simulink library "mylib"  (R2019b)
settings: Solver=VariableStepAuto  StartTime=0.0  StopTime=10.0  RelTol=1e-3
undefined symbols (not defined in the file or in its folder): AG, AH, AV, BCHL, BCHV, BG, BH, CG, CH, magnitude, Ts, XMW
libraries: $bdroot x28, TElib x2
(part 2 of 3)

== system mylib/Process Noise I=1-12 G New/TESUB6 ==
  STD : Inport
  G : Inport  Port=2
  Constant : Constant  Value=6
  Product : Product
  Subsystem : Subsystem
  Subtract : Sum  Inputs=+-
  X : Outport  VectorParamsAs1DForOutWhenUnconnected=off
  G_NEW : Outport  Port=2  VectorParamsAs1DForOutWhenUnconnected=off
  wires:
  STD/1 -> Product/2
  Product/1 -> X/1
  Subtract/1 -> Product/1
  Constant/1 -> Subtract/2
  G/1 -> Subsystem/1(G)
  Subsystem/1(TESUB7) -> Subtract/1
  Subsystem/2(G_NEW) -> G_NEW/1

== system mylib/Process Noise I=1-22/If Action Subsystem ==
  In1 : Inport
  Action Port : ActionPort
  Out1 : Outport  VectorParamsAs1DForOutWhenUnconnected=off
  wires:
  In1/1 -> Out1/1

== system mylib/Process Noise I=23-36/Gas Analysis Delay ==
  Clock : Clock
  Constant : Constant  Value=3600
  If : If  IfExpression=u1 == 0  ShowElse=off
  Math Function : Math  Operator=mod  SaturateOnIntegerOverflow=on
  Merge : Merge
  Product : Product
  Subsystem : Subsystem
      mask Display: color('Blue'), disp('MOD\nFix');
  TGAS Delay 0.1h : Constant  Value=360
  IF(TGAS) : Outport  VectorParamsAs1DForOutWhenUnconnected=off
  wires:
  Math Function/1 -> Subsystem/1(In1)
  Subsystem/2(Out2) -> Merge/2
  Subsystem/1(Out1) -> Merge/1
  Merge/1 -> If/1
  Constant/1 -> Product/2
  If/1 -> IF(TGAS)/1
  Clock/1 -> Product/1
  TGAS Delay 0.1h/1 -> Math Function/2, Subsystem/2(In2)
  Product/1 -> Math Function/1

== system mylib/Process Noise I=23-36/If Action Subsystem ==
  XCMP : Inport
  XDEL_OLD : Inport  Port=2
  XMNS : Inport  Port=3
  Action Port : ActionPort
  Add : Sum
  XDEL_NEW : Outport  VectorParamsAs1DForOutWhenUnconnected=off
  XMEAS : Outport  Port=2  VectorParamsAs1DForOutWhenUnconnected=off
  wires:
  XCMP/1 -> XDEL_NEW/1
  Add/1 -> XMEAS/1
  XDEL_OLD/1 -> Add/1
  XMNS/1 -> Add/2

== system mylib/Process Noise I=23-36/If Action Subsystem1 ==
  In1 : Inport
  Action Port : ActionPort
  Out1 : Outport  VectorParamsAs1DForOutWhenUnconnected=off
  wires:
  In1/1 -> Out1/1

== system mylib/Process Noise I=37-41/Gas Analysis Delay ==
  Clock : Clock
  Constant : Constant  Value=3600
  If : If  IfExpression=u1 == 0  ShowElse=off
  Math Function : Math  Operator=mod  SaturateOnIntegerOverflow=on
  Merge : Merge
  Product : Product
  Subsystem : Subsystem
      mask Display: color('Blue'), disp('MOD\nFix');
  TPROD Delay 0.25h : Constant  Value=900
  IF(TPROD) : Outport  VectorParamsAs1DForOutWhenUnconnected=off
  wires:
  Merge/1 -> If/1
  Subsystem/2(Out2) -> Merge/2
  Subsystem/1(Out1) -> Merge/1
  Math Function/1 -> Subsystem/1(In1)
  Constant/1 -> Product/2
  If/1 -> IF(TPROD)/1
  Clock/1 -> Product/1
  TPROD Delay 0.25h/1 -> Math Function/2, Subsystem/2(In2)
  Product/1 -> Math Function/1

== system mylib/Process Noise I=37-41/If Action Subsystem ==
  XCMP : Inport
  XDEL_OLD : Inport  Port=2
  XMNS : Inport  Port=3
  Action Port : ActionPort
  Add : Sum
  XDEL_NEW : Outport  VectorParamsAs1DForOutWhenUnconnected=off
  XMEAS : Outport  Port=2  VectorParamsAs1DForOutWhenUnconnected=off
  wires:
  XCMP/1 -> XDEL_NEW/1
  Add/1 -> XMEAS/1
  XDEL_OLD/1 -> Add/1
  XMNS/1 -> Add/2

== system mylib/Subsystem3/If Action Subsystem ==
  IDWLK : Inport
  "DIST " : Inport  Port=2
  G : Inport  Port=3
  Distrubance constants : Inport  Port=4
  Action Port : ActionPort
  Bus Creator : BusCreator  Inputs=6
  Bus Selector : BusSelector  OutputSignals=ADIST,BDIST,CDIST,DDIST,TNEXT,TLAST
  Disturbance parameters I=10-12 : Subsystem
      mask Display:
      | color('Green'), disp('Disturbance parameters\n I=10-12');
      | color('Blue');
      | port_label('input',1,'ADIST');
      | port_label('input',2,'BDIST');
      | port_label('input',3,'CDIST');
      | port_label('input',4,'DDIST');
      | port_label('input',5,'TNEXT');
      | port_label('input',6,'TLAST');
      | port_label('input',7,'IDVWLK');
      | port_label('input',8,'Distrubance constants');
      | port_label('input',9,'G');
      | port_label('output',1,'ADIST');
      | port_label('output',2,'BDIST');
      | port_label('output',3,'CDIST');
      | port_label('output',4,'DDIST');
      | port_label('output',5,'TNEXT');
      | port_label('output',6,'TLAST');
      | port_label('output',7,'G_NEW');
  DIST_NEW : Outport  PortDimensions=6  VectorParamsAs1DForOutWhenUnconnected=off
  "G_NEW " : Outport  Port=2  VectorParamsAs1DForOutWhenUnconnected=off
  wires:
  Disturbance parameters I=10-12/5("TNEXT ") -> Bus Creator/5  "TNEXT"
  Bus Creator/1 -> DIST_NEW/1
  IDWLK/1 -> Disturbance parameters I=10-12/7(IDVWLK)
  Bus Selector/1 -> Disturbance parameters I=10-12/1(ADIST)  "<ADIST>"
  Distrubance constants/1 -> Disturbance parameters I=10-12/8(Distrubance constants)
  Bus Selector/2 -> Disturbance parameters I=10-12/2(BDIST)  "<BDIST>"
  Disturbance parameters I=10-12/1("ADIST ") -> Bus Creator/1  "ADIST"
  Bus Selector/6 -> Disturbance parameters I=10-12/6(TLAST)  "<TLAST>"
  Bus Selector/5 -> Disturbance parameters I=10-12/5(TNEXT)  "<TNEXT>"
  Disturbance parameters I=10-12/4("DDIST ") -> Bus Creator/4  "DDIST"
  Disturbance parameters I=10-12/3("CDIST ") -> Bus Creator/3  "CDIST"
  Bus Selector/4 -> Disturbance parameters I=10-12/4(DDIST)  "<DDIST>"
  Disturbance parameters I=10-12/6("TLAST  ") -> Bus Creator/6  "TLAST"
  Bus Selector/3 -> Disturbance parameters I=10-12/3(CDIST)  "<CDIST>"
  "DIST "/1 -> Bus Selector/1
  Disturbance parameters I=10-12/2("BDIST ") -> Bus Creator/2  "BDIST"
  G/1 -> Disturbance parameters I=10-12/9(G)
  Disturbance parameters I=10-12/7("G_NEW ") -> "G_NEW "/1  "G_NEW"

== system mylib/Subsystem3/If Action Subsystem1 ==
  DIST_0 : Inport
  Action Port : ActionPort
  DIST : Outport  VectorParamsAs1DForOutWhenUnconnected=off
  wires:
  DIST_0/1 -> DIST/1

== system mylib/Subsystem3/Subsystem ==
  TNEXT : Inport
  Clock : Clock
  Constant : Constant  Value=3600
  Data Type Conversion : DataTypeConversion  OutDataTypeStr=double
  If : If  NumInputs=2  IfExpression=u1 == 0  ElseIfExpressions=u1 >= u2  ShowElse=off
  Product : Product
  Product1 : Product  OutDataTypeStr=fixdt(1,32,10)
  if : Outport
  elseif : Outport  Port=2
  wires:
  Data Type Conversion/1 -> If/2
  Product1/1 -> Data Type Conversion/1
  TNEXT/1 -> Product1/2
  Product/1 -> If/1
  Clock/1 -> Product/1
  Constant/1 -> Product/2, Product1/1
  If/1 -> if/1
  If/2 -> elseif/1

== system mylib/Subsystem3/Subsystem1 ==
  DIST_NEW : Inport
  Bus Creator : BusCreator  Inputs=6
  Bus Selector : BusSelector  OutputSignals=ADIST,BDIST,CDIST,DDIST,TNEXT,TLAST
  Delay{,1..5} (6 alike) : Delay  DelayLength=1  InitialCondition=0
  DIST : Outport
  wires:
  DIST_NEW/1 -> Bus Selector/1
  Bus Creator/1 -> DIST/1
  Delay/1 -> Bus Creator/1  "ADIST"
  Delay3/1 -> Bus Creator/4  "DDIST"
  Bus Selector/5 -> Delay4/1  "<TNEXT>"
  Delay4/1 -> Bus Creator/5  "TNEXT"
  Bus Selector/4 -> Delay3/1  "<DDIST>"
  Bus Selector/2 -> Delay1/1  "<BDIST>"
  Delay2/1 -> Bus Creator/3  "CDIST"
  Bus Selector/3 -> Delay2/1  "<CDIST>"
  Delay5/1 -> Bus Creator/6  "TLAST"
  Delay1/1 -> Bus Creator/2  "BDIST"
  Bus Selector/6 -> Delay5/1  "<TLAST>"
  Bus Selector/1 -> Delay/1  "<ADIST>"

== system mylib/Subsystem3/Subsystem2 ==
  In2 : Inport
  G : Inport  Port=2
  If Action Subsystem : Subsystem  TreatAsAtomicUnit=on
  If Action Subsystem1 : Subsystem  TreatAsAtomicUnit=on
  If5 : If  IfExpression=u1 == 0
  Merge : Merge
  G1 : Outport  VectorParamsAs1DForOutWhenUnconnected=off
  wires:
  In2/1 -> If Action Subsystem1/1(In1), If5/1
  If5/2 -> If Action Subsystem1/Action
  If Action Subsystem1/1(Out1) -> Merge/1
  If5/1 -> If Action Subsystem/Action
  If Action Subsystem/1(Out1) -> Merge/2
  G/1 -> If Action Subsystem/1(In1)
  Merge/1 -> G1/1

== system mylib/TESUB5/Subsystem ==
  TESUB7 : Inport
  HSPAN : Inport  Port=2
  HZERO : Inport  Port=3
  H : Sum
  Product : Product
  "H " : Outport  VectorParamsAs1DForOutWhenUnconnected=off
  wires:
  H/1 -> "H "/1
  Product/1 -> H/1
  HSPAN/1 -> Product/1
  HZERO/1 -> H/2
  TESUB7/1 -> Product/2

== system mylib/TESUB5/Subsystem1 ==
  SSPAN : Inport
  TESUB7 : Inport  Port=2
  SZERO : Inport  Port=3
  IDVFLAG : Inport  Port=4
  Product1 : Product  Inputs=3
  S1 : Sum
  "S1 " : Outport  VectorParamsAs1DForOutWhenUnconnected=off
  wires:
  SZERO/1 -> S1/2
  Product1/1 -> S1/1
  S1/1 -> "S1 "/1
  IDVFLAG/1 -> Product1/3
  TESUB7/1 -> Product1/2
  SSPAN/1 -> Product1/1

== system mylib/TESUB5/Subsystem2 ==
  TESUB7 : Inport
  SPSPAN : Inport  Port=2
  IDVFLAG : Inport  Port=3
  S1P : Product  Inputs=3
  "S1P " : Outport  VectorParamsAs1DForOutWhenUnconnected=off
  wires:
  IDVFLAG/1 -> S1P/3
  S1P/1 -> "S1P "/1
  TESUB7/1 -> S1P/2
  SPSPAN/1 -> S1P/1

== system mylib/TESUB5/Subsystem3 ==
  SP : Inport
  S1 : Inport  Port=2
  S : Inport  Port=3
  S1P : Inport  Port=4
  H : Inport  Port=5
  Add1 : Sum
  Constant : Constant  Value=3
  Constant1 : Constant  Value=2
  Divide : Product  Inputs=*/
  Math Function : Math  Operator=magnitude^2  SaturateOnIntegerOverflow=on
  Product2 : Product
  Product3 : Product
  Product4 : Product
  Subtract : Sum  Inputs=+-
  Subtract1 : Sum  Inputs=+-
  CDIST : Outport  VectorParamsAs1DForOutWhenUnconnected=off
  wires:
  Product3/1 -> Add1/2
  Subtract1/1 -> Divide/1
  Product4/1 -> Subtract1/2
  Math Function/1 -> Divide/2
  Product2/1 -> Subtract1/1
  S1/1 -> Subtract/1
  Constant/1 -> Product2/2
  SP/1 -> Product3/1
  Constant1/1 -> Product3/2
  Add1/1 -> Product4/2
  Subtract/1 -> Product2/1
  Divide/1 -> CDIST/1
  S/1 -> Subtract/2
  H/1 -> Product4/1, Math Function/1
  S1P/1 -> Add1/1

== system mylib/TESUB5/Subsystem4 ==
  SP : Inport
  S1 : Inport  Port=2
  S : Inport  Port=3
  S1P : Inport  Port=4
  H : Inport  Port=5
  Add2 : Sum
  Add3 : Sum
  Constant : Constant  Value=3
  Constant1 : Constant  Value=2
  Divide1 : Product  Inputs=*/
  Math Function1 : Math  Operator=pow  SaturateOnIntegerOverflow=on
  Product5 : Product
  Product6 : Product
  Subtract2 : Sum  Inputs=+-
  DDIST : Outport  VectorParamsAs1DForOutWhenUnconnected=off
  wires:
  Product5/1 -> Add3/1
  Divide1/1 -> DDIST/1
  SP/1 -> Add2/2
  Product6/1 -> Add3/2
  S/1 -> Subtract2/1
  Add2/1 -> Product6/2
  Math Function1/1 -> Divide1/2
  Subtract2/1 -> Product5/1
  Constant/1 -> Math Function1/2
  Add3/1 -> Divide1/1
  H/1 -> Product6/1, Math Function1/1
  S1/1 -> Subtract2/2
  S1P/1 -> Add2/1
  Constant1/1 -> Product5/2

== system mylib/TESUB5/Subsystem5 ==
  TLAST : Inport
  H : Inport  Port=2
  Add : Sum
  TNEXT : Outport  VectorParamsAs1DForOutWhenUnconnected=off
  wires:
  Add/1 -> TNEXT/1
  TLAST/1 -> Add/1
  H/1 -> Add/2

== system mylib/TESUB6/TESUB7 ==
  G : Inport
  I : Inport  Port=2
  Constant1 : Constant  Value=4294967296
  Divide : Product  Inputs=*/
  Divide1 : Product  Inputs=*/
  Gain : Gain  Gain=9228907
  New G : Math  Operator=rem  SaturateOnIntegerOverflow=on
  Product : Product
  Sum of Elements : Sum  Inputs=+
  TESUB7 : Outport  VectorParamsAs1DForOutWhenUnconnected=off
  wires:
  G/1 -> Gain/1
  Gain/1 -> New G/1
  Constant1/1 -> Divide/2, New G/2
  New G/1 -> Divide/1
  I/1 -> Divide1/2, Divide1/1
  Divide/1 -> Product/2
  Divide1/1 -> Product/1
  Product/1 -> Sum of Elements/1
  Sum of Elements/1 -> TESUB7/1

== system mylib/TESUB7/If Action Subsystem ==
  In1 : Inport
  Action Port : ActionPort
  Out1 : Outport  VectorParamsAs1DForOutWhenUnconnected=off
  wires:
  In1/1 -> Out1/1

== system mylib/TESUB7/If Action Subsystem1 ==
  In1 : Inport
  Action Port : ActionPort
  Out1 : Outport  VectorParamsAs1DForOutWhenUnconnected=off
  wires:
  In1/1 -> Out1/1

== system mylib/TESUB7 G-New/If Action Subsystem ==
  In1 : Inport
  Action Port : ActionPort
  Out1 : Outport  VectorParamsAs1DForOutWhenUnconnected=off
  wires:
  In1/1 -> Out1/1

== system mylib/TESUB7 G-New/If Action Subsystem1 ==
  In1 : Inport
  Action Port : ActionPort
  Out1 : Outport  VectorParamsAs1DForOutWhenUnconnected=off
  wires:
  In1/1 -> Out1/1

== system mylib/Valve opening limits/If Action Subsystem ==
  In1 : Inport
  Action Port : ActionPort
  Out1 : Outport  VectorParamsAs1DForOutWhenUnconnected=off
  wires:
  In1/1 -> Out1/1

== system mylib/Valve opening limits/If Action Subsystem1 ==
  In1 : Inport
  Action Port : ActionPort
  Out1 : Outport  VectorParamsAs1DForOutWhenUnconnected=off
  wires:
  In1/1 -> Out1/1

== system mylib/Valve opening limits/If Action Subsystem2 ==
  In1 : Inport
  Action Port : ActionPort
  Out1 : Outport  VectorParamsAs1DForOutWhenUnconnected=off
  wires:
  In1/1 -> Out1/1

== system mylib/Braatz Control/P Control/  ==
  DXMV : Inport
  XMV_0 : Inport  Port=2
  Add : Sum
  Delay : Delay  DelayLength=1  InitialConditionSource=Input port  InitialCondition=0
      settings: InputPortMap=u0,p4
  Subsystem1 : $bdroot/Braatz Control/Subsystem1  SystemSampleTime=-1  Latency=0  AutoFrameSizeCalculation=off
  XMV : Outport
  wires:
  XMV_0/1 -> Delay/2
  Delay/1 -> Add/1
  Add/1 -> Subsystem1/1
  Subsystem1/1 -> XMV/1, Delay/1
  DXMV/1 -> Add/2

== system mylib/Braatz Control/P Control/ERR ==
  SETPT : Inport
  XMEAS : Inport  Port=2
  High Limit : Inport  Port=3
  " " : Product  Inputs=**/
  Constant : Constant  Value=100
  Subtract : Sum  Inputs=+-
  ERR : Outport  VectorParamsAs1DForOutWhenUnconnected=off
  wires:
  Constant/1 -> " "/2
  High Limit/1 -> " "/3
  Subtract/1 -> " "/1
  SETPT/1 -> Subtract/1
  " "/1 -> ERR/1
  XMEAS/1 -> Subtract/2

== system mylib/Braatz Control/P Control/Subsystem ==
  ERR : Inport
  GAIN : Inport  Port=2
  ERROLD : Inport  Port=3
  Product : Product
  Subtract1 : Sum  Inputs=+-
  DXMV : Outport  VectorParamsAs1DForOutWhenUnconnected=off
  wires:
  GAIN/1 -> Product/1
  Product/1 -> DXMV/1
  Subtract1/1 -> Product/2
  ERROLD/1 -> Subtract1/2
  ERR/1 -> Subtract1/1

== system mylib/Braatz Control/PI Control/ERR ==
  SETPT : Inport
  XMEAS : Inport  Port=2
  High Limit : Inport  Port=3
  " " : Product  Inputs=**/
  Constant : Constant  Value=100
  Subtract : Sum  Inputs=+-
  ERR : Outport  VectorParamsAs1DForOutWhenUnconnected=off
  wires:
  Constant/1 -> " "/2
  High Limit/1 -> " "/3
  Subtract/1 -> " "/1
  XMEAS/1 -> Subtract/2
  SETPT/1 -> Subtract/1
  " "/1 -> ERR/1

== system mylib/Braatz Control/PI Control/Subsystem ==
  ERR : Inport
  GAIN : Inport  Port=2
  Sampling Interval : Inport  Port=3
  TAUI : Inport  Port=4
  ERROLD : Inport  Port=5
  Add : Sum
  DELTAT : Constant  Value=1/3600
  Product : Product
  Product1 : Product  Inputs=***/
  Subtract1 : Sum  Inputs=+-
  DXMV : Outport  VectorParamsAs1DForOutWhenUnconnected=off
  wires:
  GAIN/1 -> Product/1
  Product/1 -> DXMV/1
  ERR/1 -> Product1/1, Subtract1/1
  DELTAT/1 -> Product1/2
  Sampling Interval/1 -> Product1/3
  Subtract1/1 -> Add/1
  Product1/1 -> Add/2
  TAUI/1 -> Product1/4
  Add/1 -> Product/2
  ERROLD/1 -> Subtract1/2

== system mylib/Braatz Control/PI Control Setpoint/  ==
  DXMV : Inport
  High Limit : Inport  Port=2
  SETPT_0 : Inport  Port=3
  Add : Sum
  Constant : Constant  Value=100
  Delay : Delay  DelayLength=1  InitialConditionSource=Input port  InitialCondition=0
      settings: InputPortMap=u0,p4
  Divide : Product  Inputs=**/
  SETPT : Outport
  wires:
  Constant/1 -> Divide/3
  High Limit/1 -> Divide/2
  SETPT_0/1 -> Delay/2
  DXMV/1 -> Divide/1
  Divide/1 -> Add/2
  Delay/1 -> Add/1
  Add/1 -> Delay/1, SETPT/1

== system mylib/Braatz Control/PI Control Setpoint/ERR ==
  SETPT : Inport
  XMEAS : Inport  Port=2
  High Limit Setpoint : Inport  Port=3
  " " : Product  Inputs=**/
  Constant : Constant  Value=100
  Subtract : Sum  Inputs=+-
  ERR : Outport  VectorParamsAs1DForOutWhenUnconnected=off
  wires:
  Constant/1 -> " "/2
  High Limit Setpoint/1 -> " "/3
  Subtract/1 -> " "/1
  XMEAS/1 -> Subtract/2
  SETPT/1 -> Subtract/1
  " "/1 -> ERR/1

== system mylib/Braatz Control/PI Control Setpoint/Subsystem2 ==
  ERR : Inport
  GAIN : Inport  Port=2
  Sampling Interval : Inport  Port=3
  TAUI : Inport  Port=4
  ERROLD : Inport  Port=5
  Add : Sum
  DELTAT : Constant  Value=1/3600
  Product : Product
  Product1 : Product  Inputs=***/
  Subtract1 : Sum  Inputs=+-
  DXMV : Outport  VectorParamsAs1DForOutWhenUnconnected=off
  wires:
  GAIN/1 -> Product/1
  Product/1 -> DXMV/1
  ERR/1 -> Product1/1, Subtract1/1
  DELTAT/1 -> Product1/2
  Sampling Interval/1 -> Product1/3
  Subtract1/1 -> Add/1
  Product1/1 -> Add/2
  Add/1 -> Product/2
  TAUI/1 -> Product1/4
  ERROLD/1 -> Subtract1/2

== system mylib/Braatz Control/Sampling interval/Subsystem ==
  In1 : Inport
  In2 : Inport  Port=2
  If : If  NumInputs=2  IfExpression=u1 == u2
  If Action Subsystem : Subsystem  TreatAsAtomicUnit=on
  If Action Subsystem1 : Subsystem  TreatAsAtomicUnit=on
  Rounding Function : Rounding  Operator=round
  Out1 : Outport  VectorParamsAs1DForOutWhenUnconnected=off
  Out2 : Outport  Port=2  VectorParamsAs1DForOutWhenUnconnected=off
  wires:
  If/2 -> If Action Subsystem1/Action
  If/1 -> If Action Subsystem/Action
  In1/1 -> Rounding Function/1
  If Action Subsystem1/1(Out1) -> Out2/1
  If Action Subsystem/1(Out1) -> Out1/1
  In2/1 -> If/2
  Rounding Function/1 -> If Action Subsystem1/1(In1), If/1

== system mylib/Braatz Control/Subsystem1/If Action Subsystem ==
  In1 : Inport
  Action Port : ActionPort
  Out1 : Outport  VectorParamsAs1DForOutWhenUnconnected=off
  wires:
  In1/1 -> Out1/1

== system mylib/Braatz Control/Subsystem1/If Action Subsystem1 ==
  In1 : Inport
  Action Port : ActionPort
  Out1 : Outport  VectorParamsAs1DForOutWhenUnconnected=off
  wires:
  In1/1 -> Out1/1

== system mylib/Braatz Control/Subsystem1/If Action Subsystem2 ==
  In1 : Inport
  Action Port : ActionPort
  Out1 : Outport  VectorParamsAs1DForOutWhenUnconnected=off
  wires:
  In1/1 -> Out1/1

== system mylib/Control valve/Subsystem/If Action Subsystem ==
  XMV(I) : Inport
  Action Port : ActionPort
  VCV(I) : Outport  VectorParamsAs1DForOutWhenUnconnected=off
  wires:
  XMV(I)/1 -> VCV(I)/1

== system mylib/Control valve/Subsystem/Subsystem ==
  XMV(I) : Inport
  VCV(I) : Inport  Port=2
  IVST(I) : Inport  Port=3
  Abs : Abs
  Clock : Clock
  If : If  NumInputs=3  IfExpression=u1 == 0 | u2 > u3  ShowElse=off
  Product : Product
  Subtract : Sum  Inputs=+-
  VST(I) : Constant  Value=2
  if : Outport  VectorParamsAs1DForOutWhenUnconnected=off
  wires:
  Product/1 -> If/3
  Clock/1 -> If/1
  Abs/1 -> If/2
  IVST(I)/1 -> Product/2
  VST(I)/1 -> Product/1
  If/1 -> if/1
  VCV(I)/1 -> Subtract/1
  XMV(I)/1 -> Subtract/2
  Subtract/1 -> Abs/1

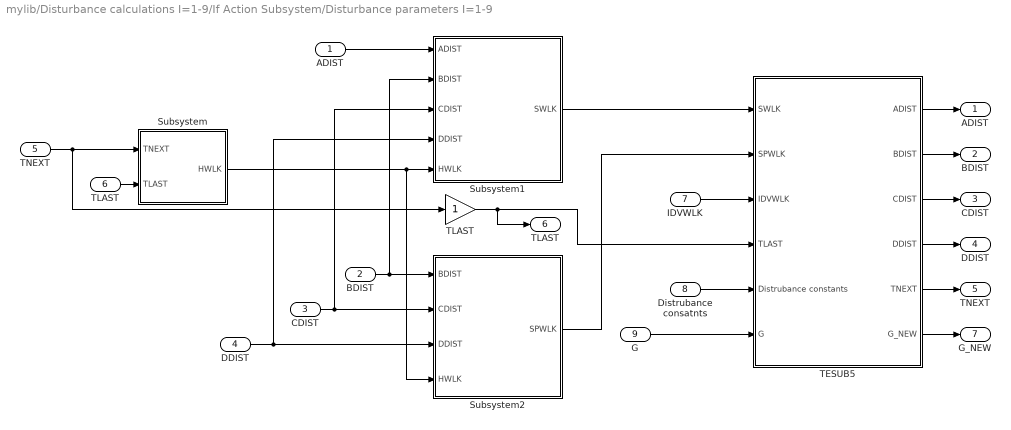
== system mylib/Disturbance calculations I=1-9/If Action Subsystem/Disturbance parameters I=1-9 ==
  ADIST : Inport
  BDIST : Inport  Port=2
  CDIST : Inport  Port=3
  DDIST : Inport  Port=4
  TNEXT : Inport  Port=5
  TLAST : Inport  Port=6
  IDVWLK : Inport  Port=7
  Distrubance consatnts : Inport  Port=8
  G : Inport  Port=9
  Subsystem : Subsystem
  Subsystem1 : Subsystem
  Subsystem2 : Subsystem
  TESUB5 : Subsystem
      mask Display:
      | color('Green'), disp('TESUB5');
      | color('Blue');
      | port_label('input',1,'SWLK');
      | port_label('input',2,'SPWLK');
      | port_label('input',3,'IDVWLK');
      | port_label('input',4,'TLAST');
      | port_label('input',5,'Disturbance constants');
      | port_label('input',6,'G');
      | port_label('output',1,'ADIST');
      | port_label('output',2,'BDIST');
      | port_label('output',3,'CDIST');
      | port_label('output',4,'DDIST');
      | port_label('output',5,'TNEXT');
      | port_label('output',6,'G_NEW');
  "TLAST " : Gain
  "ADIST " : Outport  VectorParamsAs1DForOutWhenUnconnected=off
  "BDIST " : Outport  Port=2  VectorParamsAs1DForOutWhenUnconnected=off
  "CDIST " : Outport  Port=3  VectorParamsAs1DForOutWhenUnconnected=off
  "DDIST " : Outport  Port=4  VectorParamsAs1DForOutWhenUnconnected=off
  "TNEXT " : Outport  Port=5  VectorParamsAs1DForOutWhenUnconnected=off
  "TLAST  " : Outport  Port=6  VectorParamsAs1DForOutWhenUnconnected=off
  G_NEW : Outport  Port=7  VectorParamsAs1DForOutWhenUnconnected=off
  wires:
  G/1 -> TESUB5/6(G)
  Distrubance consatnts/1 -> TESUB5/5("Distrubance constants ")
  Subsystem2/1("SPWLK ") -> TESUB5/2(SPWLK)
  Subsystem/1("HWLK ") -> Subsystem1/5(HWLK), Subsystem2/4(HWLK)
  Subsystem1/1("SWLK ") -> TESUB5/1(SWLK)
  ADIST/1 -> Subsystem1/1(ADIST)
  TLAST/1 -> Subsystem/2(TLAST)
  TESUB5/5(TNEXT) -> "TNEXT "/1
  TESUB5/4(DDIST) -> "DDIST "/1
  TESUB5/3(CDIST) -> "CDIST "/1
  TESUB5/2(BDIST) -> "BDIST "/1
  TESUB5/1(ADIST) -> "ADIST "/1
  "TLAST "/1 -> TESUB5/4(TLAST), "TLAST  "/1
  TNEXT/1 -> Subsystem/1(TNEXT), "TLAST "/1
  IDVWLK/1 -> TESUB5/3(IDVWLK)
  DDIST/1 -> Subsystem2/3(DDIST), Subsystem1/4(DDIST)
  CDIST/1 -> Subsystem2/2(CDIST), Subsystem1/3(CDIST)
  BDIST/1 -> Subsystem1/2(BDIST), Subsystem2/1(BDIST)
  TESUB5/6(G_NEW) -> G_NEW/1

== system mylib/Disturbance calculations I=1-9/Subsystem2/If Action Subsystem ==
  In1 : Inport
  Action Port : ActionPort
  Out1 : Outport  VectorParamsAs1DForOutWhenUnconnected=off
  wires:
  In1/1 -> Out1/1

== system mylib/Disturbance calculations I=1-9/Subsystem2/If Action Subsystem1 ==
  In1 : Inport
  Action Port : ActionPort
  Out1 : Outport  VectorParamsAs1DForOutWhenUnconnected=off
  wires:
  In1/1 -> Out1/1

== system mylib/Disturbance parameters I=10-12/ /If Action Subsystem ==
  In1 : Inport
  Action Port : ActionPort
  Out1 : Outport  VectorParamsAs1DForOutWhenUnconnected=off
  wires:
  In1/1 -> Out1/1

== system mylib/Disturbance parameters I=10-12/ /If Action Subsystem1 ==
  In1 : Inport
  Action Port : ActionPort
  Out1 : Outport  VectorParamsAs1DForOutWhenUnconnected=off
  wires:
  In1/1 -> Out1/1

== system mylib/Disturbance parameters I=10-12/ /Subsystem ==
  SWLK : Inport
  SPWLK : Inport  Port=2
  TLAST : Inport  Port=3
  ADIST : Gain
  Add : Sum
  BDIST : Gain
  Bus Creator : BusCreator  Inputs=5
  Constant : Constant  Value=0.1
  Subsystem : Subsystem
  Subsystem1 : Subsystem
  DIST : Outport  VectorParamsAs1DForOutWhenUnconnected=off
  wires:
  SWLK/1 -> Subsystem1/1(SWLK), Subsystem/1(SWLK), ADIST/1
  SPWLK/1 -> Subsystem1/2(SPWLK), Subsystem/2(SPWLK), BDIST/1
  ADIST/1 -> Bus Creator/1  "ADIST"
  BDIST/1 -> Bus Creator/2  "BDIST"
  Subsystem/1(CDIST) -> Bus Creator/3  "CDIST"
  Subsystem1/1(DDIST) -> Bus Creator/4  "DDIST"
  TLAST/1 -> Add/1
  Constant/1 -> Add/2
  Add/1 -> Bus Creator/5  "TNEXT"
  Bus Creator/1 -> DIST/1

== system mylib/Disturbance parameters I=10-12/ /Subsystem1 ==
  IDVWLK : Inport
  TLAST : Inport  Port=2
  Distrubance constants : Inport  Port=3
  TESUB7 : Inport  Port=4
  Add : Sum
  Bus Creator : BusCreator  Inputs=5
  Constant : Constant  Value=0.0
  Constant1 : Constant  Value=0.0
  Constant2 : Constant  Value=0.0
  Divide : Product  Inputs=*/
  HWLK : Subsystem
  Math Function : Math  Operator=magnitude^2  SaturateOnIntegerOverflow=on
  DIST : Outport  VectorParamsAs1DForOutWhenUnconnected=off
  wires:
  Bus Creator/1 -> DIST/1
  Constant/1 -> Bus Creator/1  "ADIST"
  Constant1/1 -> Bus Creator/2  "BDIST"
  Constant2/1 -> Bus Creator/4  "DDIST"
  Distrubance constants/1 -> HWLK/1(Distrubance constants)
  TLAST/1 -> Add/1
  HWLK/1(HWLK) -> Add/2, Math Function/1
  Add/1 -> Bus Creator/5  "TNEXT"
  Math Function/1 -> Divide/2
  Divide/1 -> Bus Creator/3  "CDIST"
  IDVWLK/1 -> Divide/1
  TESUB7/1 -> HWLK/2(TESUB7)

== system mylib/Enthalpy of Stream /Calculate Molar Liquid Enthalpy of stream MBtu//lb-mol/HI Enthalpy of individual components MBtu//lb ==
  T : Inport
  "     " : Product  Inputs=3
  "AH(I) Coefficient A to determine Enthalpy MBtu/lb·°F " : Constant  Value=AH
  Add : Sum  Inputs=3
  CH*T^2/3 : Subsystem
      mask Display: disp('(C×T^2)/3', 'texmode', 'on')
  Subsystem : Subsystem
      mask Display: disp('(B×T)/2', 'texmode', 'on')
  To convert °F to °C : Constant  Value=1.8
  "HI " : Outport  VectorParamsAs1DForOutWhenUnconnected=off
  wires:
  T/1 -> Subsystem/1(T), CH*T^2/3/1(T), "     "/1
  To convert °F to °C/1 -> "     "/3
  Add/1 -> "     "/2
  "AH(I) Coefficient A to determine Enthalpy MBtu/lb·°F "/1 -> Add/1
  "     "/1 -> "HI "/1
  CH*T^2/3/1(Out1) -> Add/3
  Subsystem/1(Out1) -> Add/2

== system mylib/Enthalpy of Stream /Calculate Molar Vapour Enthalpy of stream MBtu//lb-mol/HI Enthalpy of individual components MBtu//lb ==
  T : Inport
  "     " : Product  Inputs=3
  "AG(I) Coefficient A to determine Enthalpy MBtu/lb·°F " : Constant  Value=AG
  AV(I) Coefficient AV to determine Enthalpy MBtu/lb : Constant  Value=AV
  Add : Sum  Inputs=3
  Add1 : Sum  Inputs=2
  Subsystem : Subsystem
      mask Display: disp('(C×T^2)/3', 'texmode', 'on')
  Subsystem1 : Subsystem
      mask Display: disp('(B×T)/2', 'texmode', 'on')
  To convert °F to °C : Constant  Value=1.8
  "HI " : Outport  VectorParamsAs1DForOutWhenUnconnected=off
  wires:
  T/1 -> "     "/1, Subsystem1/1(T), Subsystem/1(T)
  To convert °F to °C/1 -> "     "/3
  Add/1 -> "     "/2
  "AG(I) Coefficient A to determine Enthalpy MBtu/lb·°F "/1 -> Add/1
  Add1/1 -> "HI "/1
  "     "/1 -> Add1/1
  AV(I) Coefficient AV to determine Enthalpy MBtu/lb/1 -> Add1/2
  Subsystem/1(Out1) -> Add/3
  Subsystem1/1(Out1) -> Add/2

== system mylib/Exergy/Subsystem/If Action Subsystem ==
  In1 : Inport
  Action Port : ActionPort
  Out1 : Outport  VectorParamsAs1DForOutWhenUnconnected=off
  wires:
  In1/1 -> Out1/1

== system mylib/Exergy/Subsystem2/Subsystem ==
  ITY : Inport
  Temperature of stream °C : Inport  Port=2
  XST : Inport  Port=3
  Reference Temperature : Inport  Port=4
  "Enthalpy of Stream " : $bdroot/Enthalpy of Stream   SystemSampleTime=-1  Latency=0  AutoFrameSizeCalculation=off
  Enthalpy of Stream 1 : $bdroot/Enthalpy of Stream   SystemSampleTime=-1  Latency=0  AutoFrameSizeCalculation=off
  h-h0 : Sum  Inputs=+-
  h-h0 MBtu/lb-mol : Outport  VectorParamsAs1DForOutWhenUnconnected=off
  wires:
  ITY/1 -> Enthalpy of Stream 1/1, "Enthalpy of Stream "/1
  Temperature of stream °C/1 -> "Enthalpy of Stream "/2
  "Enthalpy of Stream "/1 -> h-h0/1  "h"
  XST/1 -> Enthalpy of Stream 1/3, "Enthalpy of Stream "/3
  Reference Temperature/1 -> Enthalpy of Stream 1/2
  Enthalpy of Stream 1/1 -> h-h0/2  "h0"
  h-h0/1 -> h-h0 MBtu/lb-mol/1

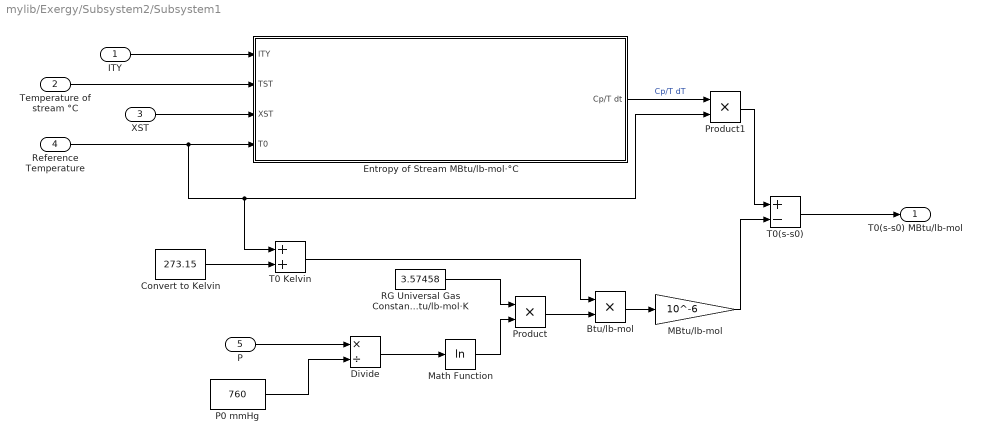
== system mylib/Exergy/Subsystem2/Subsystem1 ==
  ITY : Inport
  Temperature of stream °C : Inport  Port=2
  XST : Inport  Port=3
  Reference Temperature : Inport  Port=4
  P : Inport  Port=5
  Btu/lb-mol : Product
  Convert to Kelvin : Constant  Value=273.15
  Divide : Product  Inputs=*/
  Entropy of Stream MBtu/lb-mol·°C : Subsystem
      mask Display:
      | color('Green'), disp('TESUB1\nMolar Enthalpy of Stream\nMBtu/lb-mol');
      | color('Blue');
      | port_label('input',1,'Phase of Stream');
      | port_label('input',2,'Temperature of Stream');
      | port_label('input',3,'Composition of Stream');
      | port_label('output',1,'Enthalpy of Stream')
  MBtu/lb-mol : Gain  Gain=10^-6
  Math Function : Math  Operator=log  SaturateOnIntegerOverflow=on
  P0 mmHg : Constant  Value=760
  Product : Product
  Product1 : Product
  RG Universal Gas Constant Btu/lb-mol·K : Constant  Value=3.57458
  T0 Kelvin : Sum
  T0(s-s0) : Sum  Inputs=+-
  T0(s-s0) MBtu/lb-mol : Outport  VectorParamsAs1DForOutWhenUnconnected=off
  wires:
  ITY/1 -> Entropy of Stream MBtu/lb-mol·°C/1(ITY)
  Temperature of stream °C/1 -> Entropy of Stream MBtu/lb-mol·°C/2(TST)
  XST/1 -> Entropy of Stream MBtu/lb-mol·°C/3(XST)
  Reference Temperature/1 -> T0 Kelvin/1, Product1/2, Entropy of Stream MBtu/lb-mol·°C/4(T0)
  RG Universal Gas Constant Btu/lb-mol·K/1 -> Product/1
  Math Function/1 -> Product/2
  P/1 -> Divide/1
  P0 mmHg/1 -> Divide/2
  Divide/1 -> Math Function/1
  T0(s-s0)/1 -> T0(s-s0) MBtu/lb-mol/1
  Entropy of Stream MBtu/lb-mol·°C/1(Cp/T dt) -> Product1/1  "Cp/T dT"
  Product1/1 -> T0(s-s0)/1
  Product/1 -> Btu/lb-mol/2
  Convert to Kelvin/1 -> T0 Kelvin/2
  T0 Kelvin/1 -> Btu/lb-mol/1
  Btu/lb-mol/1 -> MBtu/lb-mol/1
  MBtu/lb-mol/1 -> T0(s-s0)/2

== system mylib/Exergy Molar Flow/Subsystem/If Action Subsystem ==
  In1 : Inport
  Action Port : ActionPort
  Out1 : Outport  VectorParamsAs1DForOutWhenUnconnected=off
  wires:
  In1/1 -> Out1/1

== system mylib/Exergy Molar Flow/Subsystem2/Subsystem ==
  ITY : Inport
  Temperature of stream °C : Inport  Port=2
  XST : Inport  Port=3
  Reference Temperature : Inport  Port=4
  "Enthalpy of Stream " : $bdroot/Enthalpy of Stream   SystemSampleTime=-1  Latency=0  AutoFrameSizeCalculation=off
  Enthalpy of Stream 1 : $bdroot/Enthalpy of Stream   SystemSampleTime=-1  Latency=0  AutoFrameSizeCalculation=off
  h-h0 : Sum  Inputs=+-
  h-h0 MBtu/lb-mol : Outport  VectorParamsAs1DForOutWhenUnconnected=off
  wires:
  h-h0/1 -> h-h0 MBtu/lb-mol/1
  Enthalpy of Stream 1/1 -> h-h0/2  "h0"
  Reference Temperature/1 -> Enthalpy of Stream 1/2
  XST/1 -> "Enthalpy of Stream "/3, Enthalpy of Stream 1/3
  "Enthalpy of Stream "/1 -> h-h0/1  "h"
  Temperature of stream °C/1 -> "Enthalpy of Stream "/2
  ITY/1 -> "Enthalpy of Stream "/1, Enthalpy of Stream 1/1

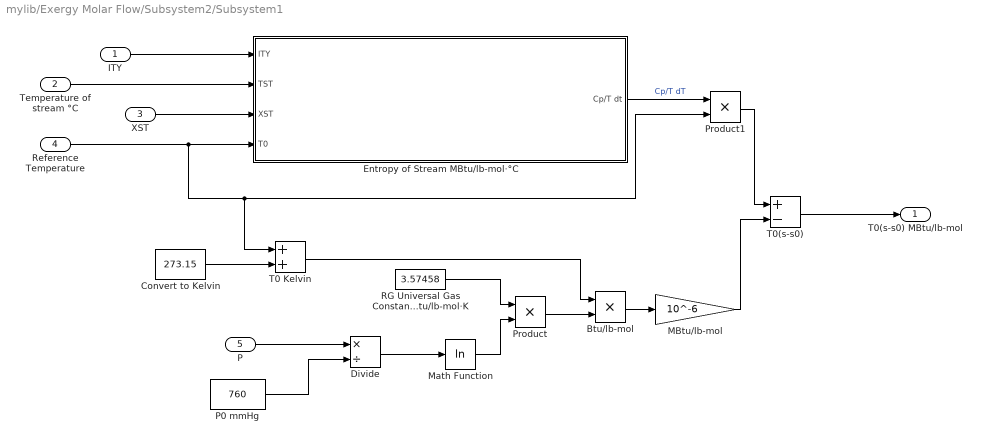
== system mylib/Exergy Molar Flow/Subsystem2/Subsystem1 ==
  ITY : Inport
  Temperature of stream °C : Inport  Port=2
  XST : Inport  Port=3
  Reference Temperature : Inport  Port=4
  P : Inport  Port=5
  Btu/lb-mol : Product
  Convert to Kelvin : Constant  Value=273.15
  Divide : Product  Inputs=*/
  Entropy of Stream MBtu/lb-mol·°C : Subsystem
      mask Display:
      | color('Green'), disp('TESUB1\nMolar Enthalpy of Stream\nMBtu/lb-mol');
      | color('Blue');
      | port_label('input',1,'Phase of Stream');
      | port_label('input',2,'Temperature of Stream');
      | port_label('input',3,'Composition of Stream');
      | port_label('output',1,'Enthalpy of Stream')
  MBtu/lb-mol : Gain  Gain=10^-6
  Math Function : Math  Operator=log  SaturateOnIntegerOverflow=on
  P0 mmHg : Constant  Value=760
  Product : Product
  Product1 : Product
  RG Universal Gas Constant Btu/lb-mol·K : Constant  Value=3.57458
  T0 Kelvin : Sum
  T0(s-s0) : Sum  Inputs=+-
  T0(s-s0) MBtu/lb-mol : Outport  VectorParamsAs1DForOutWhenUnconnected=off
  wires:
  MBtu/lb-mol/1 -> T0(s-s0)/2
  Btu/lb-mol/1 -> MBtu/lb-mol/1
  T0 Kelvin/1 -> Btu/lb-mol/1
  Convert to Kelvin/1 -> T0 Kelvin/2
  Product/1 -> Btu/lb-mol/2
  Product1/1 -> T0(s-s0)/1
  Entropy of Stream MBtu/lb-mol·°C/1(Cp/T dt) -> Product1/1  "Cp/T dT"
  T0(s-s0)/1 -> T0(s-s0) MBtu/lb-mol/1
  Divide/1 -> Math Function/1
  P0 mmHg/1 -> Divide/2
  P/1 -> Divide/1
  Math Function/1 -> Product/2
  RG Universal Gas Constant Btu/lb-mol·K/1 -> Product/1
  Reference Temperature/1 -> Entropy of Stream MBtu/lb-mol·°C/4(T0), Product1/2, T0 Kelvin/1
  XST/1 -> Entropy of Stream MBtu/lb-mol·°C/3(XST)
  Temperature of stream °C/1 -> Entropy of Stream MBtu/lb-mol·°C/2(TST)
  ITY/1 -> Entropy of Stream MBtu/lb-mol·°C/1(ITY)

== system mylib/Integration/Subsystem/If Action Subsystem ==
  Action Port : ActionPort
  Constant : Constant  Value=0
  Out1 : Outport
  wires:
  Constant/1 -> Out1/1

== system mylib/Integration/Subsystem/If Action Subsystem1 ==
  In1 : Inport
  Action Port : ActionPort
  Out1 : Outport
  wires:
  In1/1 -> Out1/1

== system mylib/Process Noise I=1-12 G New/TESUB6/Subsystem ==
  G : Inport
  Sum of Elements : Sum  Inputs=12
  TESUB7(1) : Subsystem
  TESUB7(10) : Subsystem
  TESUB7(11) : Subsystem
  TESUB7(12) : Subsystem
  TESUB7(2) : Subsystem
  TESUB7(3) : Subsystem
  TESUB7(4) : Subsystem
  TESUB7(5) : Subsystem
  TESUB7(6) : Subsystem
  TESUB7(7) : Subsystem
  TESUB7(8) : Subsystem
  TESUB7(9) : Subsystem
  TESUB7 : Outport  VectorParamsAs1DForOutWhenUnconnected=off
  G_NEW : Outport  Port=2  VectorParamsAs1DForOutWhenUnconnected=off
  wires:
  Sum of Elements/1 -> TESUB7/1
  G/1 -> TESUB7(1)/1(G)
  TESUB7(1)/2(G_NEW) -> TESUB7(2)/1(G)
  TESUB7(2)/2(G_NEW) -> TESUB7(3)/1(G)
  TESUB7(3)/2(G_NEW) -> TESUB7(4)/1(G)
  TESUB7(4)/2(G_NEW) -> TESUB7(5)/1(G)
  TESUB7(1)/1(TESUB7(1)) -> Sum of Elements/1  "TESUB7(1)"
  TESUB7(2)/1(TESUB7(2)) -> Sum of Elements/2  "TESUB7(2)"
  TESUB7(3)/1(TESUB7(3)) -> Sum of Elements/3  "TESUB7(3)"
  TESUB7(4)/1(TESUB7(4)) -> Sum of Elements/4  "TESUB7(4)"
  TESUB7(5)/1(TESUB7(5)) -> Sum of Elements/5  "TESUB7(5)"
  TESUB7(6)/1(TESUB7(6)) -> Sum of Elements/6  "TESUB7(6)"
  TESUB7(5)/2(G_NEW) -> TESUB7(6)/1(G)
  TESUB7(7)/1(TESUB7(7)) -> Sum of Elements/7  "TESUB7(7)"
  TESUB7(6)/2(G_NEW) -> TESUB7(7)/1(G)
  TESUB7(7)/2(G_NEW) -> TESUB7(8)/1(G)
  TESUB7(8)/1(TESUB7(8)) -> Sum of Elements/8  "TESUB7(8)"
  TESUB7(9)/1(TESUB7(9)) -> Sum of Elements/9  "TESUB7(9)"
  TESUB7(8)/2(G_NEW) -> TESUB7(9)/1(G)
  TESUB7(9)/2(G_NEW) -> TESUB7(10)/1(G)
  TESUB7(10)/1(TESUB7(10)) -> Sum of Elements/10  "TESUB7(10)"
  TESUB7(10)/2(G_NEW) -> TESUB7(11)/1(G)
  TESUB7(11)/1(TESUB7(11)) -> Sum of Elements/11  "TESUB7(11)"
  TESUB7(12)/1(TESUB7(12)) -> Sum of Elements/12
  TESUB7(11)/2(G_NEW) -> TESUB7(12)/1(G)
  TESUB7(12)/2(G_NEW) -> G_NEW/1

== system mylib/Process Noise I=23-36/Gas Analysis Delay/Subsystem ==
  In1 : Inport
  In2 : Inport  Port=2
  If : If  NumInputs=2  IfExpression=u1 == u2
  If Action Subsystem : Subsystem  TreatAsAtomicUnit=on
  If Action Subsystem1 : Subsystem  TreatAsAtomicUnit=on
  Rounding Function : Rounding  Operator=round
  Out1 : Outport  VectorParamsAs1DForOutWhenUnconnected=off
  Out2 : Outport  Port=2  VectorParamsAs1DForOutWhenUnconnected=off
  wires:
  If/2 -> If Action Subsystem1/Action
  If/1 -> If Action Subsystem/Action
  In1/1 -> Rounding Function/1
  If Action Subsystem1/1(Out1) -> Out2/1
  If Action Subsystem/1(Out1) -> Out1/1
  In2/1 -> If/2
  Rounding Function/1 -> If Action Subsystem1/1(In1), If/1

== system mylib/Process Noise I=37-41/Gas Analysis Delay/Subsystem ==
  In1 : Inport
  In2 : Inport  Port=2
  If : If  NumInputs=2  IfExpression=u1 == u2
  If Action Subsystem : Subsystem  TreatAsAtomicUnit=on
  If Action Subsystem1 : Subsystem  TreatAsAtomicUnit=on
  Rounding Function : Rounding  Operator=round
  Out1 : Outport  VectorParamsAs1DForOutWhenUnconnected=off
  Out2 : Outport  Port=2  VectorParamsAs1DForOutWhenUnconnected=off
  wires:
  If/2 -> If Action Subsystem1/Action
  If/1 -> If Action Subsystem/Action
  In1/1 -> Rounding Function/1
  If Action Subsystem1/1(Out1) -> Out2/1
  If Action Subsystem/1(Out1) -> Out1/1
  In2/1 -> If/2
  Rounding Function/1 -> If Action Subsystem1/1(In1), If/1

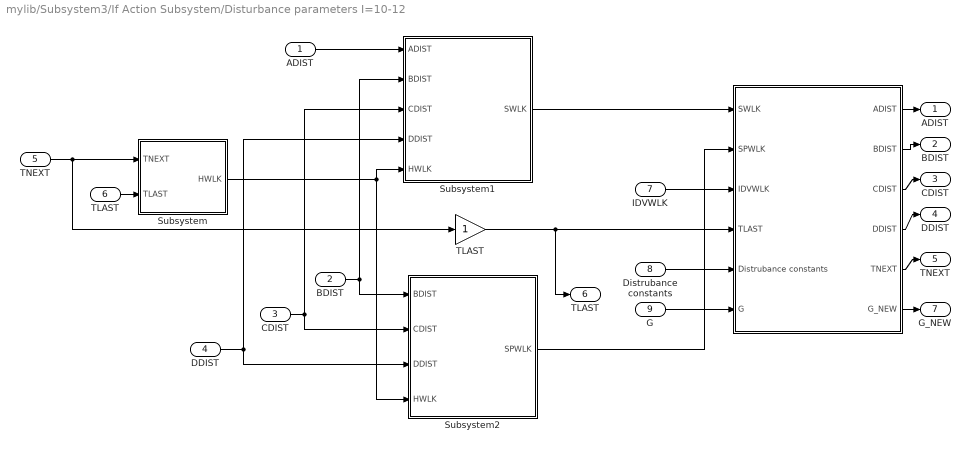
== system mylib/Subsystem3/If Action Subsystem/Disturbance parameters I=10-12 ==
  ADIST : Inport
  BDIST : Inport  Port=2
  CDIST : Inport  Port=3
  DDIST : Inport  Port=4
  TNEXT : Inport  Port=5
  TLAST : Inport  Port=6
  IDVWLK : Inport  Port=7
  Distrubance constants : Inport  Port=8
  G : Inport  Port=9
  " " : Subsystem
  Subsystem : Subsystem
  Subsystem1 : Subsystem
  Subsystem2 : Subsystem
  "TLAST " : Gain
  "ADIST " : Outport  VectorParamsAs1DForOutWhenUnconnected=off
  "BDIST " : Outport  Port=2  VectorParamsAs1DForOutWhenUnconnected=off
  "CDIST " : Outport  Port=3  VectorParamsAs1DForOutWhenUnconnected=off
  "DDIST " : Outport  Port=4  VectorParamsAs1DForOutWhenUnconnected=off
  "TNEXT " : Outport  Port=5  VectorParamsAs1DForOutWhenUnconnected=off
  "TLAST  " : Outport  Port=6  VectorParamsAs1DForOutWhenUnconnected=off
  "G_NEW " : Outport  Port=7  VectorParamsAs1DForOutWhenUnconnected=off
  wires:
  G/1 -> " "/6(G)
  Distrubance constants/1 -> " "/5(Distrubance constants)
  Subsystem2/1("SPWLK ") -> " "/2(SPWLK)
  Subsystem/1("HWLK ") -> Subsystem2/4(HWLK), Subsystem1/5(HWLK)
  Subsystem1/1("SWLK ") -> " "/1(SWLK)
  ADIST/1 -> Subsystem1/1(ADIST)
  TLAST/1 -> Subsystem/2(TLAST)
  " "/5(TNEXT) -> "TNEXT "/1
  " "/4(DDIST) -> "DDIST "/1
  " "/3(CDIST) -> "CDIST "/1
  " "/2(BDIST) -> "BDIST "/1
  " "/1(ADIST) -> "ADIST "/1
  "TLAST "/1 -> " "/4(TLAST), "TLAST  "/1
  TNEXT/1 -> Subsystem/1(TNEXT), "TLAST "/1
  IDVWLK/1 -> " "/3(IDVWLK)
  DDIST/1 -> Subsystem2/3(DDIST), Subsystem1/4(DDIST)
  CDIST/1 -> Subsystem2/2(CDIST), Subsystem1/3(CDIST)
  BDIST/1 -> Subsystem1/2(BDIST), Subsystem2/1(BDIST)
  " "/6(G_NEW) -> "G_NEW "/1

== system mylib/Subsystem3/Subsystem2/If Action Subsystem ==
  In1 : Inport
  Action Port : ActionPort
  Out1 : Outport  VectorParamsAs1DForOutWhenUnconnected=off
  wires:
  In1/1 -> Out1/1

== system mylib/Subsystem3/Subsystem2/If Action Subsystem1 ==
  In1 : Inport
  Action Port : ActionPort
  Out1 : Outport  VectorParamsAs1DForOutWhenUnconnected=off
  wires:
  In1/1 -> Out1/1

== system mylib/Braatz Control/Sampling interval/Subsystem/If Action Subsystem ==
  Action Port : ActionPort
  Constant : Constant  Value=0
  Out1 : Outport  VectorParamsAs1DForOutWhenUnconnected=off
  wires:
  Constant/1 -> Out1/1

== system mylib/Braatz Control/Sampling interval/Subsystem/If Action Subsystem1 ==
  In1 : Inport
  Action Port : ActionPort
  Out1 : Outport  VectorParamsAs1DForOutWhenUnconnected=off
  wires:
  In1/1 -> Out1/1

== system mylib/Disturbance calculations I=1-9/If Action Subsystem/Disturbance parameters I=1-9/Subsystem ==
  TNEXT : Inport
  TLAST : Inport  Port=2
  HWLK : Sum  Inputs=+-
  "HWLK " : Outport  VectorParamsAs1DForOutWhenUnconnected=off
  wires:
  HWLK/1 -> "HWLK "/1
  TLAST/1 -> HWLK/2
  TNEXT/1 -> HWLK/1

== system mylib/Disturbance calculations I=1-9/If Action Subsystem/Disturbance parameters I=1-9/Subsystem1 ==
  ADIST : Inport
  BDIST : Inport  Port=2
  CDIST : Inport  Port=3
  DDIST : Inport  Port=4
  HWLK : Inport  Port=5
  Add : Sum
  Add1 : Sum
  Product : Product
  Product1 : Product
  Product2 : Product
  SWLK : Sum
  "SWLK " : Outport  VectorParamsAs1DForOutWhenUnconnected=off
  wires:
  HWLK/1 -> Product/1, Product1/1, Product2/1
  Add1/1 -> Product2/2
  Product1/1 -> Add1/1
  DDIST/1 -> Product/2
  Product2/1 -> SWLK/2
  Add/1 -> Product1/2
  Product/1 -> Add/1
  SWLK/1 -> "SWLK "/1
  CDIST/1 -> Add/2
  ADIST/1 -> SWLK/1
  BDIST/1 -> Add1/2

== system mylib/Disturbance calculations I=1-9/If Action Subsystem/Disturbance parameters I=1-9/Subsystem2 ==
  BDIST : Inport
  CDIST : Inport  Port=2
  DDIST : Inport  Port=3
  HWLK : Inport  Port=4
  Add2 : Sum
  Constant : Constant  Value=3
  Constant1 : Constant  Value=2
  Product3 : Product  Inputs=3
  Product4 : Product
  Product5 : Product
  SPWLK : Sum
  "SPWLK " : Outport  VectorParamsAs1DForOutWhenUnconnected=off
  wires:
  BDIST/1 -> SPWLK/1
  CDIST/1 -> Product4/2
  Constant1/1 -> Product4/1
  Product3/1 -> Add2/1
  HWLK/1 -> Product3/2, Product5/1
  Product5/1 -> SPWLK/2
  Constant/1 -> Product3/1
  Add2/1 -> Product5/2
  SPWLK/1 -> "SPWLK "/1
  Product4/1 -> Add2/2
  DDIST/1 -> Product3/3

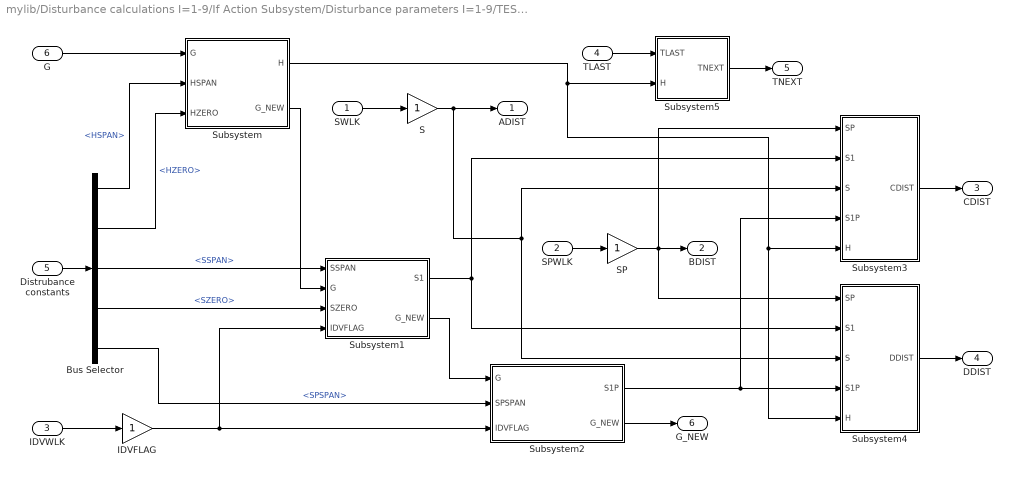
== system mylib/Disturbance calculations I=1-9/If Action Subsystem/Disturbance parameters I=1-9/TESUB5 ==
  SWLK : Inport
  SPWLK : Inport  Port=2
  IDVWLK : Inport  Port=3
  TLAST : Inport  Port=4
  "Distrubance constants " : Inport  Port=5
  G : Inport  Port=6
  Bus Selector : BusSelector  OutputSignals=HSPAN,HZERO,SSPAN,SZERO,SPSPAN
  IDVFLAG : Gain
  S : Gain
  SP : Gain
  Subsystem : Subsystem
  Subsystem1 : Subsystem
  Subsystem2 : Subsystem
  Subsystem3 : Subsystem
  Subsystem4 : Subsystem
  Subsystem5 : Subsystem
  ADIST : Outport  VectorParamsAs1DForOutWhenUnconnected=off
  BDIST : Outport  Port=2  VectorParamsAs1DForOutWhenUnconnected=off
  CDIST : Outport  Port=3  VectorParamsAs1DForOutWhenUnconnected=off
  DDIST : Outport  Port=4  VectorParamsAs1DForOutWhenUnconnected=off
  TNEXT : Outport  Port=5  VectorParamsAs1DForOutWhenUnconnected=off
  G_NEW : Outport  Port=6  VectorParamsAs1DForOutWhenUnconnected=off
  wires:
  Bus Selector/2 -> Subsystem/3(HZERO)  "<HZERO>"
  "Distrubance constants "/1 -> Bus Selector/1
  Bus Selector/5 -> Subsystem2/2(SPSPAN)  "<SPSPAN>"
  Bus Selector/1 -> Subsystem/2(HSPAN)  "<HSPAN>"
  Bus Selector/3 -> Subsystem1/1(SSPAN)  "<SSPAN>"
  Bus Selector/4 -> Subsystem1/3(SZERO)  "<SZERO>"
  Subsystem5/1(TNEXT) -> TNEXT/1
  TLAST/1 -> Subsystem5/1(TLAST)
  Subsystem4/1(DDIST) -> DDIST/1
  Subsystem3/1(CDIST) -> CDIST/1
  Subsystem2/1("S1P ") -> Subsystem4/4(S1P), Subsystem3/4(S1P)
  Subsystem1/1("S1 ") -> Subsystem4/2(S1), Subsystem3/2(S1)
  Subsystem/1("H ") -> Subsystem4/5(H), Subsystem3/5(H), Subsystem5/2(H)
  SP/1 -> Subsystem3/1(SP), BDIST/1, Subsystem4/1(SP)
  S/1 -> Subsystem3/3(S), Subsystem4/3(S), ADIST/1
  SPWLK/1 -> SP/1
  SWLK/1 -> S/1
  IDVFLAG/1 -> Subsystem2/3(IDVFLAG), Subsystem1/4(IDVFLAG)
  IDVWLK/1 -> IDVFLAG/1
  G/1 -> Subsystem/1(G)
  Subsystem/2(G_NEW) -> Subsystem1/2(G)
  Subsystem1/2(G_NEW) -> Subsystem2/1(G)
  Subsystem2/2(G_NEW) -> G_NEW/1

== system mylib/Disturbance parameters I=10-12/ /Subsystem/Subsystem ==
  SWLK : Inport
  SPWLK : Inport  Port=2
  Add : Sum
  Constant : Constant  Value=3
  Constant1 : Constant  Value=0.2
  Constant2 : Constant  Value=0.01
  Divide : Product  Inputs=*/
  Product : Product
  Product1 : Product
  Unary Minus : UnaryMinus
  CDIST : Outport  VectorParamsAs1DForOutWhenUnconnected=off
  wires:
  Constant/1 -> Product/1
  Constant1/1 -> Product1/1
  SWLK/1 -> Product/2
  SPWLK/1 -> Product1/2
  Product/1 -> Add/1
  Product1/1 -> Add/2
  Add/1 -> Unary Minus/1
  Unary Minus/1 -> Divide/1
  Constant2/1 -> Divide/2
  Divide/1 -> CDIST/1

== system mylib/Disturbance parameters I=10-12/ /Subsystem/Subsystem1 ==
  SWLK : Inport
  SPWLK : Inport  Port=2
  Add : Sum
  Constant : Constant  Value=2
  Constant1 : Constant  Value=0.1
  Constant2 : Constant  Value=0.001
  Divide : Product  Inputs=*/
  Product : Product
  Product1 : Product
  DDIST : Outport  VectorParamsAs1DForOutWhenUnconnected=off
  wires:
  Constant/1 -> Product/1
  Constant1/1 -> Product1/1
  SWLK/1 -> Product/2
  SPWLK/1 -> Product1/2
  Product/1 -> Add/1
  Product1/1 -> Add/2
  Add/1 -> Divide/1
  Constant2/1 -> Divide/2
  Divide/1 -> DDIST/1

== system mylib/Disturbance parameters I=10-12/ /Subsystem1/HWLK ==
  Distrubance constants : Inport
  TESUB7 : Inport  Port=2
  Add : Sum
  Bus Selector : BusSelector  OutputSignals=HSPAN,HZERO
  Product : Product
  HWLK : Outport  VectorParamsAs1DForOutWhenUnconnected=off
  wires:
  Distrubance constants/1 -> Bus Selector/1
  TESUB7/1 -> Product/1
  Bus Selector/1 -> Product/2  "<HSPAN>"
  Product/1 -> Add/1
  Bus Selector/2 -> Add/2  "<HZERO>"
  Add/1 -> HWLK/1

== system mylib/Enthalpy of Stream /Calculate Molar Liquid Enthalpy of stream MBtu//lb-mol/HI Enthalpy of individual components MBtu//lb/CH*T^2//3 ==
  T : Inport
  "   " : Constant  Value=3
  "        " : Product  Inputs=**/
  CH(I) Coefficient C to determine Enthalpy MBtu/lb·°F³ : Constant  Value=CH
  Math Function : Math  Operator=magnitude^2  SaturateOnIntegerOverflow=on
  Out1 : Outport  VectorParamsAs1DForOutWhenUnconnected=off
  wires:
  Math Function/1 -> "        "/2
  "        "/1 -> Out1/1
  CH(I) Coefficient C to determine Enthalpy MBtu/lb·°F³/1 -> "        "/1
  T/1 -> Math Function/1
  "   "/1 -> "        "/3

== system mylib/Enthalpy of Stream /Calculate Molar Liquid Enthalpy of stream MBtu//lb-mol/HI Enthalpy of individual components MBtu//lb/Subsystem ==
  T : Inport
  "  " : Constant  Value=2
  "         " : Product  Inputs=**/
  BH(I) Coefficient B to determine Enthalpy MBtu/lb·°F² : Constant  Value=BH
  Out1 : Outport  VectorParamsAs1DForOutWhenUnconnected=off
  wires:
  "  "/1 -> "         "/3
  BH(I) Coefficient B to determine Enthalpy MBtu/lb·°F²/1 -> "         "/1
  "         "/1 -> Out1/1
  T/1 -> "         "/2

== system mylib/Enthalpy of Stream /Calculate Molar Vapour Enthalpy of stream MBtu//lb-mol/HI Enthalpy of individual components MBtu//lb/Subsystem ==
  T : Inport
  "   " : Constant  Value=3
  "        " : Product  Inputs=**/
  CG(I) Coefficient C to determine Enthalpy MBtu/lb·°F³ : Constant  Value=CG
  Math Function : Math  Operator=magnitude^2  SaturateOnIntegerOverflow=on
  Out1 : Outport  VectorParamsAs1DForOutWhenUnconnected=off
  wires:
  "   "/1 -> "        "/3
  "        "/1 -> Out1/1
  Math Function/1 -> "        "/2
  CG(I) Coefficient C to determine Enthalpy MBtu/lb·°F³/1 -> "        "/1
  T/1 -> Math Function/1

== system mylib/Enthalpy of Stream /Calculate Molar Vapour Enthalpy of stream MBtu//lb-mol/HI Enthalpy of individual components MBtu//lb/Subsystem1 ==
  T : Inport
  "  " : Constant  Value=2
  "         " : Product  Inputs=**/
  BG(I) Coefficient B to determine Enthalpy MBtu/lb·°F² : Constant  Value=BG
  Out1 : Outport  VectorParamsAs1DForOutWhenUnconnected=off
  wires:
  "  "/1 -> "         "/3
  BG(I) Coefficient B to determine Enthalpy MBtu/lb·°F²/1 -> "         "/1
  "         "/1 -> Out1/1
  T/1 -> "         "/2

== system mylib/Exergy/Subsystem2/Subsystem1/Entropy of Stream MBtu//lb-mol·°C ==
  ITY : Inport
  TST : Inport  Port=2
  XST : Inport  Port=3
  T0 : Inport  Port=4
  If : If  IfExpression=u1 == 0
  If Action Subsystem : Subsystem  TreatAsAtomicUnit=on
  If Action Subsystem2 : Subsystem  TreatAsAtomicUnit=on
  Molar Entropy change of stream MBtu/lb-mol·°C : Merge
  Molar Liquid Entropy change of stream MBtu/lb-mol·°C : Subsystem
  Molar Vapour Entropy change of stream MBtu/lb-mol·°C : Subsystem
  Cp/T dt : Outport  VectorParamsAs1DForOutWhenUnconnected=off
  wires:
  Molar Entropy change of stream MBtu/lb-mol·°C/1 -> Cp/T dt/1
  If Action Subsystem/1(Out1) -> Molar Entropy change of stream MBtu/lb-mol·°C/1
  If/2 -> If Action Subsystem2/Action
  If Action Subsystem2/1(Out1) -> Molar Entropy change of stream MBtu/lb-mol·°C/2
  Molar Liquid Entropy change of stream MBtu/lb-mol·°C/1(Cp/T dt) -> If Action Subsystem/1(In1)
  ITY/1 -> If/1
  If/1 -> If Action Subsystem/Action
  XST/1 -> Molar Vapour Entropy change of stream MBtu/lb-mol·°C/2(XST(I,1)), Molar Liquid Entropy change of stream MBtu/lb-mol·°C/2(XST(I,1))
  TST/1 -> Molar Vapour Entropy change of stream MBtu/lb-mol·°C/1(T), Molar Liquid Entropy change of stream MBtu/lb-mol·°C/1(T)
  Molar Vapour Entropy change of stream MBtu/lb-mol·°C/1(Cp/T dt) -> If Action Subsystem2/1(In1)
  T0/1 -> Molar Liquid Entropy change of stream MBtu/lb-mol·°C/3(T0), Molar Vapour Entropy change of stream MBtu/lb-mol·°C/3(T0)

== system mylib/Exergy Molar Flow/Subsystem2/Subsystem1/Entropy of Stream MBtu//lb-mol·°C ==
  ITY : Inport
  TST : Inport  Port=2
  XST : Inport  Port=3
  T0 : Inport  Port=4
  If : If  IfExpression=u1 == 0
  If Action Subsystem : Subsystem  TreatAsAtomicUnit=on
  If Action Subsystem2 : Subsystem  TreatAsAtomicUnit=on
  Molar Entropy change of stream MBtu/lb-mol·°C : Merge
  Molar Liquid Entropy change of stream MBtu/lb-mol·°C : Subsystem
  Molar Vapour Entropy change of stream MBtu/lb-mol·°C : Subsystem
  Cp/T dt : Outport  VectorParamsAs1DForOutWhenUnconnected=off
  wires:
  T0/1 -> Molar Vapour Entropy change of stream MBtu/lb-mol·°C/3(T0), Molar Liquid Entropy change of stream MBtu/lb-mol·°C/3(T0)
  Molar Vapour Entropy change of stream MBtu/lb-mol·°C/1(Cp/T dt) -> If Action Subsystem2/1(In1)
  TST/1 -> Molar Liquid Entropy change of stream MBtu/lb-mol·°C/1(T), Molar Vapour Entropy change of stream MBtu/lb-mol·°C/1(T)
  XST/1 -> Molar Liquid Entropy change of stream MBtu/lb-mol·°C/2(XST(I,1)), Molar Vapour Entropy change of stream MBtu/lb-mol·°C/2(XST(I,1))
  If/1 -> If Action Subsystem/Action
  ITY/1 -> If/1
  Molar Liquid Entropy change of stream MBtu/lb-mol·°C/1(Cp/T dt) -> If Action Subsystem/1(In1)
  If Action Subsystem2/1(Out1) -> Molar Entropy change of stream MBtu/lb-mol·°C/2
  If/2 -> If Action Subsystem2/Action
  If Action Subsystem/1(Out1) -> Molar Entropy change of stream MBtu/lb-mol·°C/1
  Molar Entropy change of stream MBtu/lb-mol·°C/1 -> Cp/T dt/1

== system mylib/Process Noise I=1-12 G New/TESUB6/Subsystem/TESUB7(1) ==
  G : Inport
  I : Constant
  TESUB7 : $bdroot/TESUB7 G-New  SystemSampleTime=-1  Latency=0  AutoFrameSizeCalculation=off
  TESUB7(1) : Outport  VectorParamsAs1DForOutWhenUnconnected=off
  G_NEW : Outport  Port=2  VectorParamsAs1DForOutWhenUnconnected=off
  wires:
  I/1 -> TESUB7/1
  TESUB7/2 -> G_NEW/1
  G/1 -> TESUB7/2
  TESUB7/1 -> TESUB7(1)/1

== system mylib/Process Noise I=1-12 G New/TESUB6/Subsystem/TESUB7(10) ==
  G : Inport
  I : Constant  Value=10
  TESUB7 : $bdroot/TESUB7 G-New  SystemSampleTime=-1  Latency=0  AutoFrameSizeCalculation=off
  TESUB7(10) : Outport  VectorParamsAs1DForOutWhenUnconnected=off
  G_NEW : Outport  Port=2  VectorParamsAs1DForOutWhenUnconnected=off
  wires:
  I/1 -> TESUB7/1
  TESUB7/2 -> G_NEW/1
  G/1 -> TESUB7/2
  TESUB7/1 -> TESUB7(10)/1

== system mylib/Process Noise I=1-12 G New/TESUB6/Subsystem/TESUB7(11) ==
  G : Inport
  I : Constant  Value=11
  TESUB7 : $bdroot/TESUB7 G-New  SystemSampleTime=-1  Latency=0  AutoFrameSizeCalculation=off
  TESUB7(11) : Outport  VectorParamsAs1DForOutWhenUnconnected=off
  G_NEW : Outport  Port=2  VectorParamsAs1DForOutWhenUnconnected=off
  wires:
  I/1 -> TESUB7/1
  TESUB7/2 -> G_NEW/1
  G/1 -> TESUB7/2
  TESUB7/1 -> TESUB7(11)/1

== system mylib/Process Noise I=1-12 G New/TESUB6/Subsystem/TESUB7(12) ==
  G : Inport
  I : Constant  Value=12
  TESUB7 : $bdroot/TESUB7 G-New  SystemSampleTime=-1  Latency=0  AutoFrameSizeCalculation=off
  TESUB7(12) : Outport  VectorParamsAs1DForOutWhenUnconnected=off
  G_NEW : Outport  Port=2  VectorParamsAs1DForOutWhenUnconnected=off
  wires:
  I/1 -> TESUB7/1
  TESUB7/2 -> G_NEW/1
  G/1 -> TESUB7/2
  TESUB7/1 -> TESUB7(12)/1

== system mylib/Process Noise I=1-12 G New/TESUB6/Subsystem/TESUB7(2) ==
  G : Inport
  I : Constant  Value=2
  TESUB7 : $bdroot/TESUB7 G-New  SystemSampleTime=-1  Latency=0  AutoFrameSizeCalculation=off
  TESUB7(2) : Outport  VectorParamsAs1DForOutWhenUnconnected=off
  G_NEW : Outport  Port=2  VectorParamsAs1DForOutWhenUnconnected=off
  wires:
  I/1 -> TESUB7/1
  TESUB7/2 -> G_NEW/1
  G/1 -> TESUB7/2
  TESUB7/1 -> TESUB7(2)/1
